simulink model "rtwdemo_advsc"  (Simulink 6.0)
settings: Solver=FixedStepDiscrete  StartTime=0.0  StopTime=10.0  RelTol=1e-3
PostLoadFcn:
  | open_system('rtwdemo_advsc/Auto');
values from neighbouring files (symbols this model uses):
  LOWER = Simulink.Parameter    [rtwdemo_exprfolding_data.m]
  T1Break = Simulink.Parameter    [rtwdemo_exprfolding_data.m]    (also in rtwdemo_paraminline_data.m)
  T1Data = Simulink.Parameter    [rtwdemo_exprfolding_data.m]    (also in rtwdemo_paraminline_data.m)
  T2Data = Simulink.Parameter    [rtwdemo_exprfolding_data.m]    (also in rtwdemo_paraminline_data.m)
  UPPER = Simulink.Parameter    [rtwdemo_exprfolding_data.m]
undefined symbols (not defined in the file or in its folder): K1
libraries: rtwdemowidgets x3
settings Model: CovMetricSettings=d  Creator=The MathWorks Inc.  LastModifiedBy=batserve  ExtModeAutoUpdateStatusClock=off
settings DataIOCC: SaveOutput=off  SaveTime=off  SignalLoggingName=sigsOut
settings OptimizationCC: InlineParams=on  EnforceIntegerDowncast=off  StateBitsets=on  DataBitsets=on  UseTempVars=on
settings DebuggingCC: CheckExecutionContextPreStartOutputMsg=on  CheckExecutionContextRuntimeOutputMsg=on  SignalResolutionControl=UseLocalSettings  SolverPrmCheckMsg=none
settings RTWCC: TLCOptions=-p0  GenerateReport=on  RTWVerbose=off  ProcessScript=grt_make_rtw_hook  LaunchReport=on
settings CodeAppCC: ForceParamTrailComments=on  PrefixModelToSubsysFcnNames=off

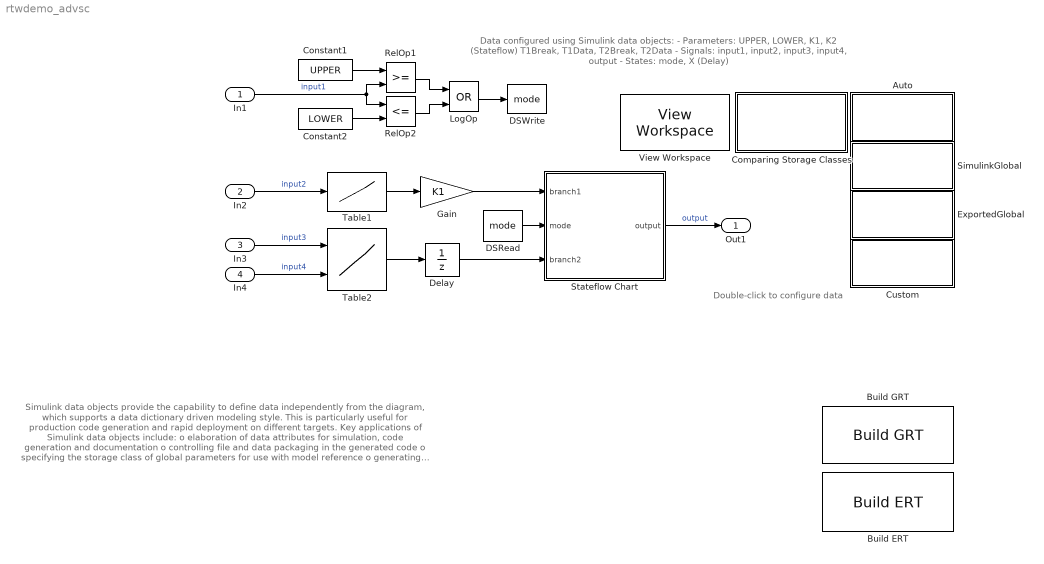
== system rtwdemo_advsc ==
  note: Double-click to configure data
  note: Data configured using Simulink data objects:
      | - Parameters: UPPER, LOWER, K1, K2 (Stateflow)
      |   T1Break, T1Data, T2Break, T2Data
      | - Signals: input1, input2, input3, input4, output
      | - States: mode, X (Delay)
  note: Simulink data objects provide the capability to define data independently from the
      | diagram, which supports a data dictionary driven modeling style.  This is particularly
      | useful for production code generation and rapid deployment on different targets.
      |
      | Key applications of Simulink data objects include:
      | o elaboration of data attributes for simulation, code generation and documentation
      | o controlling file and data packaging in the generated code
      | o specifying the storage class of global parameters for use with model reference
      | o generating ASAP2 and other calibration data files
      |
      | This model illustrates the use of built-in and custom storage classes.
      | Real-Time Workshop supports built-in storage classes.  Custom storage
      | classes require a Real-Time Workshop Embedded Coder license.
  In1 : Inport  Port=1  PortDimensions=1  SampleTime=1  LatchInput=off
  In2 : Inport  Port=2  PortDimensions=1  LatchInput=off
  In3 : Inport  Port=3  PortDimensions=1  LatchInput=off
  In4 : Inport  Port=4  PortDimensions=1  LatchInput=off
  Auto : Subsystem  PropExecContextAcrossSSBoundary=on  mask(Advanced data packaging - create data){StorageClass=Auto, DataInitFcn=rtwdemo_advsc_init}
      mask help: OpenFcn creates data with the specified storage class for data packaging demo.
      mask init:
      | dispStr = 'Initialize data with\nStorageClass: ';
      | dispStr = [dispStr, StorageClass];
      settings: OpenFcn=feval(get_param(gcb, 'DataInitFcn'), get_param(gcb, 'StorageClass'));
      mask StyleString: popup(Auto|SimulinkGlobal|ExportedGlobal|Custom),edit
      mask Display: disp([StorageClass, '\nStorage Class']);
  Build ERT : rtwdemowidgets/Build ERT  attrib_overrides={}
  Build GRT : rtwdemowidgets/Build GRT  attrib_overrides={}
  Comparing Storage Classes : Subsystem  PropExecContextAcrossSSBoundary=on
      mask Display: disp(['Compare the\noptions ..', '.\n(double-click)']);
  Constant1 : Constant  Value=UPPER
  Constant2 : Constant  Value=LOWER
  Custom : Subsystem  PropExecContextAcrossSSBoundary=on  mask(Advanced data packaging - create data){StorageClass=Custom, DataInitFcn=rtwdemo_advsc_init}
      mask help: OpenFcn creates data with the specified storage class for data packaging demo.
      mask init:
      | dispStr = 'Initialize data with\nStorageClass: ';
      | dispStr = [dispStr, StorageClass];
      settings: OpenFcn=feval(get_param(gcb, 'DataInitFcn'), get_param(gcb, 'StorageClass'));
      mask StyleString: popup(Auto|SimulinkGlobal|ExportedGlobal|Custom),edit
      mask Display: disp([StorageClass, '\nStorage Class']);
  DSRead : DataStoreRead  DialogController=Simulink.DDGSource  DataStoreName=mode  SampleTime=1
  DSWrite : DataStoreWrite  DialogController=Simulink.DDGSource  DataStoreName=mode  SampleTime=-1
  Delay : UnitDelay  StateIdentifier=X  StateMustResolveToSignalObject=on
  ExportedGlobal : Subsystem  PropExecContextAcrossSSBoundary=on  mask(Advanced data packaging - create data){StorageClass=ExportedGlobal, DataInitFcn=rtwdemo_advsc_init}
      mask help: OpenFcn creates data with the specified storage class for data packaging demo.
      mask init:
      | dispStr = 'Initialize data with\nStorageClass: ';
      | dispStr = [dispStr, StorageClass];
      settings: OpenFcn=feval(get_param(gcb, 'DataInitFcn'), get_param(gcb, 'StorageClass'));
      mask StyleString: popup(Auto|SimulinkGlobal|ExportedGlobal|Custom),edit
      mask Display: disp([StorageClass, '\nStorage Class']);
  Gain : Gain  Gain=K1  SaturateOnIntegerOverflow=on
  LogOp : Logic  Operator=OR
  RelOp1 : RelationalOperator  InputSameDT=on
  RelOp2 : RelationalOperator  Operator=<=  InputSameDT=on
  SimulinkGlobal : Subsystem  PropExecContextAcrossSSBoundary=on  mask(Advanced data packaging - create data){StorageClass=SimulinkGlobal, DataInitFcn=rtwdemo_advsc_init}
      mask help: OpenFcn creates data with the specified storage class for data packaging demo.
      mask init:
      | dispStr = 'Initialize data with\nStorageClass: ';
      | dispStr = [dispStr, StorageClass];
      settings: OpenFcn=feval(get_param(gcb, 'DataInitFcn'), get_param(gcb, 'StorageClass'));
      mask StyleString: popup(Auto|SimulinkGlobal|ExportedGlobal|Custom),edit
      mask Display: disp([StorageClass, '\nStorage Class']);
  Stateflow Chart : Stateflow chart  PropExecContextAcrossSSBoundary=on
      settings: PermitHierarchicalResolution=ParametersOnly
  Table1 : Lookup  DialogController=Simulink.DDGSource  InputValues=T1Break  OutputValues=T1Data  SaturateOnIntegerOverflow=on
  Table2 : Lookup2D  DialogController=Simulink.DDGSource  RowIndex=T2Break  ColumnIndex=T2Break  OutputValues=T2Data  OutScaling=2^-10  InputSameDT=on
  View Workspace : rtwdemowidgets/View Workspace
  Out1 : Outport
  wires:
  RelOp1/1 -> LogOp/1
  RelOp2/1 -> LogOp/2
  Constant2/1 -> RelOp2/2
  In2/1 -> Table1/1  "input2"
  Gain/1 -> Stateflow Chart/1(branch1)
  Table1/1 -> Gain/1
  Table2/1 -> Delay/1
  Constant1/1 -> RelOp1/1
  In1/1 -> RelOp1/2, RelOp2/1  "input1"
  In3/1 -> Table2/1  "input3"
  In4/1 -> Table2/2  "input4"
  Stateflow Chart/1(output) -> Out1/1  "output"
  Delay/1 -> Stateflow Chart/3(branch2)
  LogOp/1 -> DSWrite/1
  DSRead/1 -> Stateflow Chart/2(mode)

== system rtwdemo_advsc/Auto ==

== system rtwdemo_advsc/Comparing Storage Classes ==
  note: NOTE: All descriptions assume that the inline parameters and signal storage reuse optimizations are ON.
  note: 1. Auto storage class:
      |
      | Motivation:
      | - Maximize efficiency of the generated code
      |
      | Behavior:
      | - Parameters are inlined and intermediate signals are eliminated
      | - All states and root-level I/O are members of persistent data structures
      |
      | Advantages:
      | - Optimized code generation
      | - Default behavior when optimizations enabled (easy to use)
      |
      | Disadvantages:
      | - Parameters and signals do not appear as variables in the generated code
  note: 2. SimulinkGlobal storage class:
      |
      | Motivation:
      | - Provide visibility (persistence) for selected data
      |
      | Behavior:
      | - Select parameters and signals are members of persistent data structures
      | - All states and root-level I/O are members of persistent data structures
      |
      | Advantages:
      | - Only increase memory usage for data of interest
      | - Provides visibility to data without limiting modeling flexibility and code efficiency
      |
      | Disadvantages:
      | - Minimal control over variable names
  note: 3. Unstructured storage classes (e.g., ExportedGlobal):
      |
      | Motivation:
      | - Interface to global data in hand-written (legacy) code
      |
      | Behavior:
      | - Select parameters and signals are global, unstructured variables
      | - Select states and root-level I/O are global, unstructured variables
      |
      | Advantages:
      | - Data names are preserved in the generated code
      |
      | Disadvantages:
      | - Imposes certain modeling restrictions
      | - Disables certain code optimizations
  note: 4. Custom storage classes (CSCs):
      |
      | Motivation:
      | - Generate custom (user-defined) data packaging to conform with
      |     virtually any legacy data packaging and development process
      |
      | Behavior:
      | - Representation determined by custom storage class definitions
      |
      | Advantages:
      | - Full control over location, packaging and format of data
      | - Control over comments and pragmas (compiler directives)
      |
      | Disadvantages:
      | - Imposes certain modeling restrictions
      | - Disables certain code optimizations

== system rtwdemo_advsc/Custom ==

== system rtwdemo_advsc/ExportedGlobal ==

== system rtwdemo_advsc/SimulinkGlobal ==

== stateflow chart Stateflow Chart ==
  note: This chart is acting as an if-else condition,
      |     with the result multiplied by K2.
      | Using a Simulink switch (or if-action) and gain block,
      |     results in virtually identical code.
  (junction 7) -> (junction 4) : {output = branch1;}
  (junction 4) -> (junction 6) : {output *= K2;}
  (junction 5) -> (junction 4) : {output = branch2;}
  (default) -> (junction 5)
  (junction 5) -> (junction 7) : [mode]
  data: branch1 input double size=1; mode input boolean size=1; branch2 input double size=1; output output double size=1; K2 parameter double size=1
